simulink model "asbCubeSat"  (R2020a)
settings: Solver=ode3  StartTime=0.0  StopTime=86400*365.25*1  FixedStep=CubeSatTimeStep  RelTol=1e-3  EnableMultiTasking=on
PreLoadFcn:
  | if ~builtin('license','test','Virtual_Reality_Toolbox')
  |     assignin('base','variantVisualization',0)
  | end
PostLoadFcn:
  | ATM_Model=3 %
InitFcn:
  | if evalin('base', 'exist(''variantVisualization'',''var'')') && ...
  |         evalin('base', 'variantVisualization == 1')
  |     if ~builtin('license','checkout','Virtual_Reality_Toolbox')
  |         error(message('aeroblks_cubesat:cubesat:licenseFailAnim'));
  |     end
  | end
  | 
  | if ~evalin('base','exist(''CubeSatTimeStep'')')
  |     assignin('base','CubeSatTimeStep',1);
  | end
StopFcn:
  | %save('./work/simulation/alt_km_simulation.mat','alt_km_simulation','-v7.3')
  | 
  | save( ['./work/simulation/alt_km_simulation','_a_',get_param('asbCubeSat/Edit Initial Orbit and Attitude', 'a'), '_Area_', sprintf('%.4f',vehicle.Area),'.mat'],'alt_km_simulation','-v7.3')
undefined symbols (not defined in the file): CubeSatTimeStep, initCond, magnitude, Solar_Activity, vehicle
libraries: aerolibutil x12, aerolibatmos2 x6, aerolibconvert2 x3, simulink x2, asbCubeSatEnvironmentLib x1, SignalEditorBlockLib x1, sharedutil x1, asbCubeSatActuatorsLib x1, asbCubeSatSensorsLib x1, asbCubeSatDynamicsLib x1, asbCubeSatFSWLib x1, aerolibobsolete x1
(part 1 of 2)
settings Model: RequirementInfo={} %GIDa_aedc6be2_fb6a_446c_8c25_10b8bc9db182  SimulationMode=accelerator  SnapshotInterval=1  ExtModeAutoUpdateStatusClock=off  OrderedModelArguments=off  Creator=The MathWorks, Inc.  LastModifiedBy=ge49gar
settings SolverCC: AutoInsertRateTranBlk=on
settings DataIOCC: LimitDataPoints=on  SaveFormat=Array  SaveOutput=off  DSMLogging=off  SaveTime=off  ReturnWorkspaceOutputs=off
settings OptimizationCC: DefaultParameterBehavior=Inlined  OptimizeBlockIOStorage=off  BufferReuse=off  GlobalBufferReuse=off  ExpressionFolding=off  ExpressionDepthLimit=2147483647  LocalBlockOutputs=off  InitFltsAndDblsToZero=on  LifeSpan=inf  OptimizeDataStoreBuffers=off  BusAssignmentInplaceUpdate=off
settings DebuggingCC: SignalResolutionControl=TryResolveAllWithWarning  MultiTaskDSMMsg=warning  MultiTaskCondExecSysMsg=none  AssertControl=DisableAll  StateNameClashWarn=warning  PregeneratedLibrarySubsystemCodeDiagnostic=none  SFUnexpectedBacktrackingDiag=warning  SFNoUnconditionalDefaultTransitionDiag=warning  SFExecutionAtInitializationDiag=none  ArithmeticOperatorsInVariantConditions=warning
settings HardwareCC: ProdBitPerPointer=32  ProdBitPerSizeT=32  ProdBitPerPtrDiffT=32  ProdLargestAtomicFloat=None  ProdIntDivRoundTo=Undefined  ProdEndianess=Unspecified  ProdWordSize=32  ProdHWDeviceType=32-bit Generic
settings ModelReferenceCC: UpdateModelReferenceTargets=IfOutOfDate  ModelReferenceMinAlgLoopOccurrences=on  PropagateSignalLabelsOutOfModel=off
settings SFSimCC: SimUseLocalCustomCode=off
settings RTWCC: RTWUseLocalCustomCode=off
settings CodeAppCC: StateflowObjectComments=on
settings GRTTargetCC: TargetFcnLib=ansi_tfl_tmw.mat  TargetLangStandard=C89/C90 (ANSI)  CombineOutputUpdateFcns=off  GRTInterface=on
settings ConfigComp: CovMetricSettings=dw  CovHtmlReporting=on  CovSaveCumulativeToWorkspaceVar=on  CovSaveSingleToWorkspaceVar=on  CovExternalEMLEnable=off

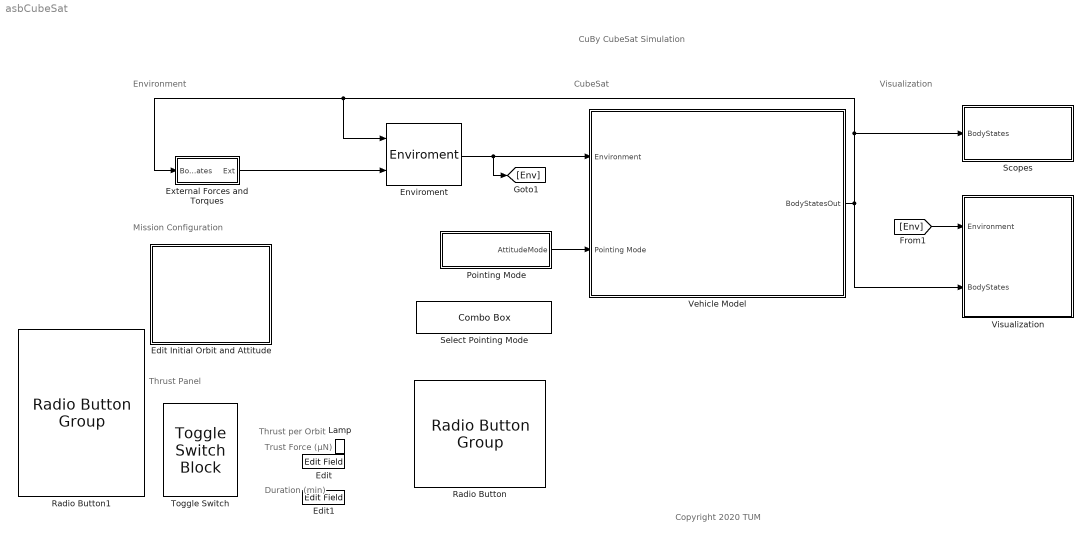
== system asbCubeSat ==
  note: Duration (min)
  note: Trust Force (µN)
  note: Thrust per Orbit
  note: Thrust Panel
  note: Visualization
  note: CubeSat
  note: Environment
  note: Copyright 2020 TUM
  note: CuBy CubeSat Simulation
  note: Mission Configuration
  Edit : EditField  LabelPosition=Hide  ShowInitialText=on  Alignment=Center
  Edit Initial Orbit and Attitude : Subsystem  mask(CubeSat Initial Conditions){sim_t0=2458928.8744, epoch=2452637.5, method=Keplerian Orbital Elements, a=6740285, ecc=0.1, incl=96.89, omega=337.5, argp=93.4872, nu=302.9234, truelon=0, arglat=0, lonper=0, r_eci=[4533222.8936 -2365511.728 3729499.3489], v_eci=[-5234.4767 1366.6412 6128.4254], r_ecef=[4811340.466 1709232.8008 3739578.4636], v_ecef=[-4446.0927 -3269.5147 6116.7671], lla=[36.4038927 19.5576255 -41750.4973], v_ned=[8059.0526 -1592.5303 622.75621], euler=[0 0 0], pqr=[0 0 -0.05168], dAT=37, dUT1=-0.1193, pm=[2.141e-05 6.93e-05], dCIP=[1.014e-07 -6.81e-08], lod=0}
      mask prompts: sim_t0 "aeroblks_cubesat:cubesat:StartDate"; epoch "aeroblks_cubesat:cubesat:ECIEpoch"; method "aeroblks_cubesat:cubesat:InputMethod"; a "aeroblks_cubesat:cubesat:SemiMajorAxis"; ecc "aeroblks_cubesat:cubesat:Eccentricity"; incl "aeroblks_cubesat:cubesat:Inclination"; omega "aeroblks_cubesat:cubesat:RAAN"; argp "aeroblks_cubesat:cubesat:ArgP"; nu "aeroblks_cubesat:cubesat:TrueAnomaly"; truelon "aeroblks_cubesat:cubesat:TrueLon"; arglat "aeroblks_cubesat:cubesat:ArgLat"; lonper "aeroblks_cubesat:cubesat:LonPer"; r_eci "aeroblks_cubesat:cubesat:ECIPos"; v_eci "aeroblks_cubesat:cubesat:ECIVel"; r_ecef "aeroblks_cubesat:cubesat:ECEFPos"; v_ecef "aeroblks_cubesat:cubesat:ECEFVel"; lla "aeroblks_cubesat:cubesat:LLA"; v_ned "aeroblks_cubesat:cubesat:NEDVel"; euler "aeroblks_cubesat:cubesat:Euler"; pqr "aeroblks_cubesat:cubesat:BodyAngRates"; dAT "aeroblks_cubesat:cubesat:dTAI"; dUT1 "aeroblks_cubesat:cubesat:DUT1"; pm "aeroblks_cubesat:cubesat:DPolar"; dCIP "aeroblks_cubesat:cubesat:DCIP"; lod "aeroblks_cubesat:cubesat:DLOD"
      mask help: aeroblks_cubesat:cubesat:InitCondBlockDesc
      mask init:
      | initCond = cubeSatCallback(gcb, 'computeIC', method, sim_t0, epoch, a, ecc, incl,...
      |     omega, argp, nu, truelon, arglat, lonper, r_eci, v_eci, r_ecef, v_ecef, lla,...
      |     v_ned, euler, pqr, dAT, dUT1, pm, dCIP, lod);
      mask TypeOptions method: aeroblks_cubesat:cubesat:InputKeplerian | aeroblks_cubesat:cubesat:InputECI | aeroblks_cubesat:cubesat:InputECEF | aeroblks_cubesat:cubesat:InputLLANED
      mask Callback method: cubeSatCallback(gcb, 'handleMethod');
      mask Callback ecc: cubeSatCallback(gcb, 'handleCircularOrbit');
      mask Callback incl: cubeSatCallback(gcb, 'handleCircularOrbit');
      mask DialogControl sim_t0 Prompt: Start date [Julian date]:
      mask DialogControl sim_t0 Tooltip: aeroblks_cubesat:cubesat:StartDateTT
      mask DialogControl icTab Prompt: aeroblks_cubesat:cubesat:InitCond
      mask DialogControl epoch Prompt: Epoch of ECI frame [Julian date]:
      mask DialogControl epoch Tooltip: aeroblks_cubesat:cubesat:ECIEpochTT
      mask DialogControl Container9 Prompt: aeroblks_cubesat:cubesat:InitCondOrbit
      mask DialogControl method Prompt: Input method:
      mask DialogControl method Tooltip: aeroblks_cubesat:cubesat:InputMethodTT
      mask DialogControl a Prompt: Semi-major axis [m]:
      mask DialogControl a Tooltip: aeroblks_cubesat:cubesat:SemiMajorAxisTT
      mask DialogControl ecc Prompt: Eccentricity:
      mask DialogControl ecc Tooltip: aeroblks_cubesat:cubesat:EccentricityTT
      mask DialogControl incl Prompt: Inclination [deg]:
      mask DialogControl incl Tooltip: aeroblks_cubesat:cubesat:InclinationTT
      mask DialogControl omega Prompt: Right ascension of the ascending node [deg]:
      mask DialogControl omega Tooltip: aeroblks_cubesat:cubesat:RAANTT
      mask DialogControl argp Prompt: Argument of periapsis [deg]:
      mask DialogControl argp Tooltip: aeroblks_cubesat:cubesat:ArgPTT
      mask DialogControl nu Prompt: True anomaly [deg]:
      mask DialogControl nu Tooltip: aeroblks_cubesat:cubesat:TrueAnomalyTT
      mask DialogControl truelon Prompt: True longitude [deg] (circular equatorial):
      mask DialogControl truelon Tooltip: aeroblks_cubesat:cubesat:TrueLonTT
      mask DialogControl arglat Prompt: Argument of latitude [deg] (circular inclined):
      mask DialogControl arglat Tooltip: aeroblks_cubesat:cubesat:ArgLatTT
      mask DialogControl lonper Prompt: Longitude of periapsis [deg] (elliptical equatorial):
      mask DialogControl lonper Tooltip: aeroblks_cubesat:cubesat:LonPerTT
      mask DialogControl r_eci Prompt: ECI position vector [m]:
      mask DialogControl r_eci Tooltip: aeroblks_cubesat:cubesat:ECIPosTT
      mask DialogControl v_eci Prompt: ECI velocity vector [m/s]:
      mask DialogControl v_eci Tooltip: aeroblks_cubesat:cubesat:ECIVelTT
      mask DialogControl r_ecef Prompt: ECEF position vector [m]:
      mask DialogControl r_ecef Tooltip: aeroblks_cubesat:cubesat:ECEFPosTT
      mask DialogControl v_ecef Prompt: ECEF velocity vector [m/s]:
      mask DialogControl v_ecef Tooltip: aeroblks_cubesat:cubesat:ECEFVelTT
      mask DialogControl lla Prompt: Geodetic latitude, longitude, altitude [deg, deg, m]:
      mask DialogControl lla Tooltip: aeroblks_cubesat:cubesat:LLATT
      mask DialogControl v_ned Prompt: NED velocity vector [m/s]:
      mask DialogControl v_ned Tooltip: aeroblks_cubesat:cubesat:NEDVelTT
      mask DialogControl Container11 Prompt: aeroblks_cubesat:cubesat:InitCondAttitude
      mask DialogControl euler Prompt: <html>Initial Euler angles (roll, pitch, yaw) [deg]:</html>
      mask DialogControl euler Tooltip: aeroblks_cubesat:cubesat:EulerTT
      mask DialogControl pqr Prompt: Initial body angular rates [deg/s]:
      mask DialogControl pqr Tooltip: aeroblks_cubesat:cubesat:BodyAngRatesTT
      mask DialogControl epTab Prompt: aeroblks_cubesat:cubesat:EOPTab
      mask DialogControl dAT Prompt: Difference between TAI and UTC [sec]:
      mask DialogControl dAT Tooltip: aeroblks_cubesat:cubesat:dTAITT
      mask DialogControl dUT1 Prompt: Difference between UTC and UT1 [sec]:
      mask DialogControl dUT1 Tooltip: aeroblks_cubesat:cubesat:DUT1TT
      mask DialogControl pm Prompt: Polar displacement [deg deg]:
      mask DialogControl pm Tooltip: aeroblks_cubesat:cubesat:DPolarTT
      mask DialogControl dCIP Prompt: CIP adjustment [deg deg]:
      mask DialogControl dCIP Tooltip: aeroblks_cubesat:cubesat:DCIPTT
      mask DialogControl lod Prompt: Excess length of day [sec]:
      mask DialogControl lod Tooltip: aeroblks_cubesat:cubesat:DLODTT
      mask Display:
      | text(.1, .9, [' a = ' sprintf('%.1f', str2double(get_param(gcb, 'a'))) ' m'],'horizontalAlignment','left','texmode','on');
      | text(.1, .75, [' e = ' get_param(gcb, 'ecc')],'horizontalAlignment','left','texmode', 'on')
      | text(.1, .6, ['  i = ' get_param(gcb, 'incl') '\circ'],'horizontalAlignment','left','texmode', 'on')
      | text(.1, .45, ['\Omega = ' get_param(gcb, 'omega') '\circ'],'horizontalAlignment','left','texmode', 'on')
      | text(.1, .3, ['\omega = ' get_param(gcb, 'argp') '\circ'],'horizontalAlignment','left','texmode', 'on')
      | text(.1, .15, [' \nu = ' get_param(gcb, 'nu') '\circ'],'horizontalAlignment','left','texmode', 'on')
  Edit1 : EditField  LabelPosition=Hide  ShowInitialText=on  Alignment=Center
  Enviroment : asbCubeSatEnvironmentLib/Enviroment  SystemSampleTime=-1  Latency=0  AutoFrameSizeCalculation=off
  External Forces and Torques : Subsystem
  Lamp : LampBlock  LabelPosition=Hide
  Pointing Mode : Subsystem
  Radio Button : RadioButtonGroup  LabelPosition=Hide  SelectedLabel=NRLMSISE-00 + F10.7 & Ap  ButtonGroupName=Atmospheric Model
      settings: Values={{'No Drag', 'ISA', 'NRLMSISE-00', 'NRLMSISE-00 + F10.7 & Ap'}, [0 1 2 3]}
  Radio Button1 : RadioButtonGroup  ButtonGroupName=Group
      settings: Values={{'Label1', 'Label2', 'Label3'}, [0 1 2]}
  Scopes : Subsystem  VariantControl=visOff
  Select Pointing Mode : ComboBox  LabelPosition=Hide  SelectedLabel=Nadir Pointing (Earth)
      settings: Values={{'Standby', 'Nadir Pointing (Earth)', 'Sun Tracking', 'Custom Schedule'}, [0 1 2 3]}
  Toggle Switch : ToggleSwitchBlock
      settings: Values={{'Off', 'On'}, [0 1]}
  Vehicle Model : Subsystem
      mask Display: image('CubeSatVehicle.PNG');
  Visualization : Subsystem  Variant=on  mask(Set Animation Properties){visSampleTime=5, cubesatSize=2e5, showAntenna=on, antennaHeight=1e6, antennaHalfAngle=25}
      mask prompts: visSampleTime "aeroblks_cubesat:cubesat:AnimSampleTime"; cubesatSize "aeroblks_cubesat:cubesat:MdlSize"; showAntenna "aeroblks_cubesat:cubesat:ShowCone"; antennaHeight "aeroblks_cubesat:cubesat:ConeHeight"; antennaHalfAngle "aeroblks_cubesat:cubesat:ConeAngle"
      mask help: aeroblks_cubesat:cubesat:VisBlockDesc
      mask Callback showAntenna:
      | if evalin('base', 'exist(''variantVisualization'',''var'')') ...
      |     && evalin('base', 'variantVisualization == 1') ...
      |     && builtin('license','test','Virtual_Reality_Toolbox')
      | 
      |     enable = get_param(gcb,'MaskEnables');
      |     if strcmp(get_param(gcb, 'showAntenna'), 'off')
      |         enable(4:5) = {'off'};
      |     else
      |         enable(4:5) = {'on'};
      |     end
      |     set_param(gcb,'MaskEnables', enable);
      |     clear enable
      | end
      mask DialogControl vrOpenBtn Prompt: aeroblks_cubesat:cubesat:AnimOpenBtn
      mask DialogControl vrOpenBtn Callback:
      | if builtin('license','checkout','Virtual_Reality_Toolbox')
      |     vrmfunc('FnOpen',getSimulinkBlockHandle([gcb '/Virtual Reality World/VR Sink']));
      | end
      mask DialogControl visSampleTime Prompt: Animation refresh rate:
      mask DialogControl visSampleTime Tooltip: aeroblks_cubesat:cubesat:AnimSampleTimeTT
      mask DialogControl cubesatSize Prompt: CubeSat display size [m]:
      mask DialogControl cubesatSize Tooltip: aeroblks_cubesat:cubesat:MdlSizeTT
      mask DialogControl Container3 Prompt: aeroblks_cubesat:cubesat:AntennaPropArea
      mask DialogControl showAntenna Prompt: Show antenna cone in animation
      mask DialogControl showAntenna Tooltip: aeroblks_cubesat:cubesat:ShowConeTT
      mask DialogControl antennaHeight Prompt: Antenna cone height [m]:
      mask DialogControl antennaHeight Tooltip: aeroblks_cubesat:cubesat:ConeHeightTT
      mask DialogControl antennaHalfAngle Prompt: Antenna cone half angle [deg]:
      mask DialogControl antennaHalfAngle Tooltip: aeroblks_cubesat:cubesat:ConeAngleTT
  wires:
  Enviroment/1 -> [Env], Vehicle Model/1(Environment)
  External Forces and Torques/1(Ext) -> Enviroment/2
  Vehicle Model/1(BodyStatesOut) -> Visualization/2(BodyStates), Scopes/1(BodyStates), External Forces and Torques/1(BodyStates), Enviroment/1
  Pointing Mode/1(AttitudeMode) -> Vehicle Model/2(Pointing Mode)
  [Env] -> Visualization/1(Environment)

== system asbCubeSat/Edit Initial Orbit and Attitude ==

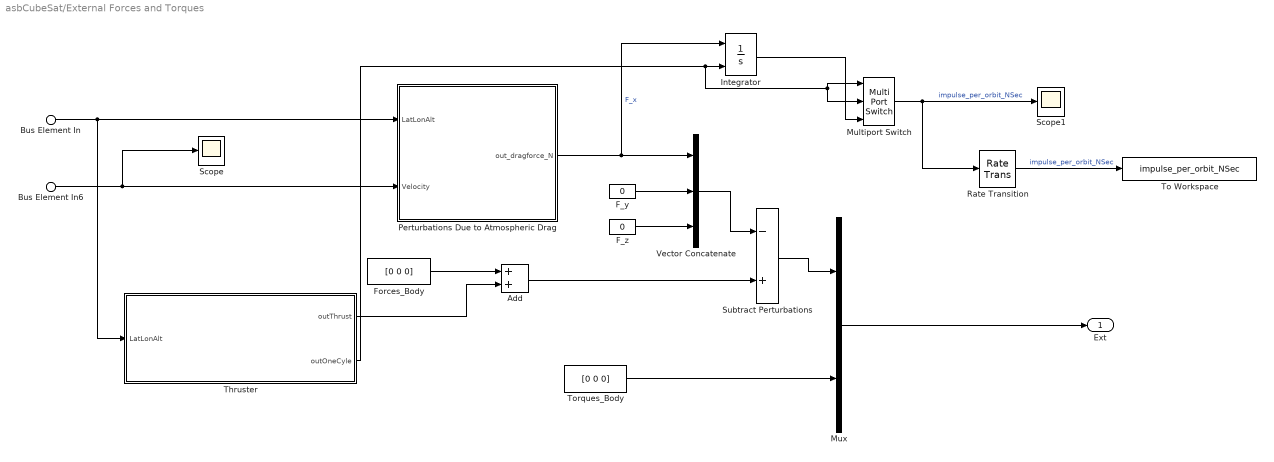
== system asbCubeSat/External Forces and Torques ==
  Bus Element In : Inport  PortName=BodyStates  Element=LatLonAlt
  Bus Element In6 : Inport  PortName=BodyStates  Element=V_ecef
  Add : Sum
  F_y : Constant  Value=0
  F_z : Constant  Value=0
  Forces_Body : Constant  Value=[0 0 0]
  Integrator : Integrator  ExternalReset=falling
  Multiport Switch : MultiPortSwitch  DataPortOrder=Zero-based contiguous  Inputs=2  zeroidx=on
  Mux : Mux  RequirementInfo={} %GIDa_ef4ca723_4eef_40f8_bb1e_99de60d2b248  Inputs=2
  Perturbations Due to Atmospheric Drag : Subsystem
  Rate Transition : RateTransition  OutPortSampleTime=60
  Scope : Scope
  Scope1 : Scope
  "Subtract Perturbations " : Sum  Inputs=-+
  Thruster : Subsystem
  To Workspace : ToWorkspace  VariableName=impulse_per_orbit_NSec  SaveFormat=Structure With Time  SampleTime=-1
  Torques_Body : Constant  Value=[0 0 0]
  Vector Concatenate : Concatenate  NumInputs=3
  Ext : Outport  RequirementInfo={} %GIDa_0f078eca_6127_499d_b81c_658503a40261  VectorParamsAs1DForOutWhenUnconnected=off
  wires:
  Forces_Body/1 -> Add/1
  Torques_Body/1 -> Mux/2
  Mux/1 -> Ext/1
  "Subtract Perturbations "/1 -> Mux/1
  Perturbations Due to Atmospheric Drag/1(out_dragforce_N) -> Integrator/1, Vector Concatenate/1  "F_x"
  Vector Concatenate/1 -> "Subtract Perturbations "/1
  F_y/1 -> Vector Concatenate/2
  F_z/1 -> Vector Concatenate/3
  Bus Element In/1 -> Thruster/1(LatLonAlt), Perturbations Due to Atmospheric Drag/1(LatLonAlt)
  Bus Element In6/1 -> Scope/1, Perturbations Due to Atmospheric Drag/2(Velocity)
  Thruster/1(outThrust) -> Add/2
  Add/1 -> "Subtract Perturbations "/2
  Thruster/2(outOneCyle) -> Multiport Switch/2, Multiport Switch/1, Integrator/2
  Integrator/1 -> Multiport Switch/3
  Multiport Switch/1 -> Scope1/1, Rate Transition/1  "impulse_per_orbit_NSec"
  Rate Transition/1 -> To Workspace/1  "impulse_per_orbit_NSec"

== system asbCubeSat/Pointing Mode ==
  note: Modes:
      | 0 = Off
      | 1 = Earth (Nadir)
      | 2 = Sun
  Mode : Constant  SampleTime=-1
  Multiport Switch : MultiPortSwitch  DataPortOrder=Specify indices  DataPortIndices={3, [0,1,2]}  DiagnosticForDefault=None
  Signal Editor : SignalEditorBlockLib/Signal Editor  FileName=SignalEditorPointing.mat  ActiveScenario=PointingScenario  ActiveSignal=PointingMode  IsBus=off  OutputBusObjectStr=Bus: BusObject  SampleTime=0  Interpolate=off  ZeroCross=off  OutputAfterFinalValue=Setting to zero  Unit=inherit  PreserveSignalName=on
  AttitudeMode : Outport  VectorParamsAs1DForOutWhenUnconnected=off
  wires:
  Signal Editor/1 -> Multiport Switch/2
  Mode/1 -> Multiport Switch/1, Multiport Switch/3
  Multiport Switch/1 -> AttitudeMode/1

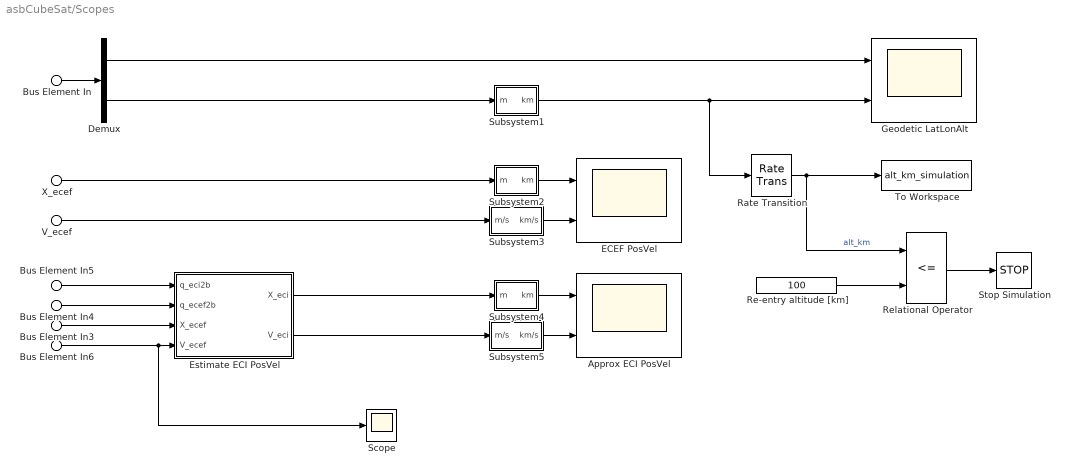
== system asbCubeSat/Scopes ==
  Bus Element In : Inport  PortName=BodyStates  Element=LatLonAlt
  X_ecef : Inport  PortName=BodyStates  Element=X_ecef
  Bus Element In3 : Inport  PortName=BodyStates  Element=X_ecef
  V_ecef : Inport  PortName=BodyStates  Element=V_ecef
  Bus Element In6 : Inport  PortName=BodyStates  Element=V_ecef
  Bus Element In4 : Inport  PortName=BodyStates  Element=q_ecef2b
  Bus Element In5 : Inport  PortName=BodyStates  Element=q_eci2b
  Approx ECI PosVel : Scope  NumInputPorts=2
  Demux : Demux  Outputs=[2 1]
  ECEF PosVel : Scope  NumInputPorts=2
  Estimate ECI PosVel : Subsystem
  Geodetic LatLonAlt : Scope  NumInputPorts=2
  Rate Transition : RateTransition  OutPortSampleTime=60
  Re-entry altitude [km] : Constant  Value=100
  Relational Operator : RelationalOperator  Operator=<=  OutDataTypeStr=boolean  RndMeth=Simplest
  Scope : Scope
  Stop Simulation : Stop
  Subsystem1 : Subsystem
  Subsystem2 : Subsystem
  Subsystem3 : Subsystem
  Subsystem4 : Subsystem
  Subsystem5 : Subsystem
  To Workspace : ToWorkspace  VariableName=alt_km_simulation  SaveFormat=Structure With Time  SampleTime=-1
  wires:
  Bus Element In/1 -> Demux/1
  Demux/1 -> Geodetic LatLonAlt/1
  Demux/2 -> Subsystem1/1(m)
  X_ecef/1 -> Subsystem2/1(m)
  V_ecef/1 -> Subsystem3/1(m/s)
  Estimate ECI PosVel/1(X_eci) -> Subsystem4/1(m)
  Estimate ECI PosVel/2(V_eci) -> Subsystem5/1(m/s)
  Bus Element In5/1 -> Estimate ECI PosVel/1(q_eci2b)
  Bus Element In4/1 -> Estimate ECI PosVel/2(q_ecef2b)
  Bus Element In3/1 -> Estimate ECI PosVel/3(X_ecef)
  Subsystem1/1(km) -> Rate Transition/1, Geodetic LatLonAlt/2
  Subsystem2/1(km) -> ECEF PosVel/1
  Subsystem3/1(km/s) -> ECEF PosVel/2
  Subsystem4/1(km) -> Approx ECI PosVel/1
  Subsystem5/1(km/s) -> Approx ECI PosVel/2
  Bus Element In6/1 -> Scope/1, Estimate ECI PosVel/4(V_ecef)
  Rate Transition/1 -> Relational Operator/1, To Workspace/1  "alt_km"
  Relational Operator/1 -> Stop Simulation/1
  Re-entry altitude [km]/1 -> Relational Operator/2

== system asbCubeSat/Vehicle Model ==
  note: Flight Software
  note: Plant Model
  Environment : Inport
  Pointing Mode : Inport  Port=2
  Vehicle Control Actuators : asbCubeSatActuatorsLib/Vehicle Control Actuators  SystemSampleTime=-1  Latency=0  AutoFrameSizeCalculation=off
  Vehicle Control Sensors : asbCubeSatSensorsLib/Vehicle Control Sensors  SystemSampleTime=-1  Latency=0  AutoFrameSizeCalculation=off
  Vehicle Dynamics : asbCubeSatDynamicsLib/Vehicle Dynamics  SystemSampleTime=-1  Latency=0  AutoFrameSizeCalculation=off
  Vehicle Flight Software : asbCubeSatFSWLib/Vehicle Flight Software  SystemSampleTime=-1  Latency=0  AutoFrameSizeCalculation=off
  BodyStatesOut : Outport  OutDataTypeStr=Bus: StatesOutBus  VectorParamsAs1DForOutWhenUnconnected=off
  wires:
  Vehicle Dynamics/1 -> Vehicle Control Sensors/1, BodyStatesOut/1
  Pointing Mode/1 -> Vehicle Flight Software/1
  Vehicle Control Sensors/1 -> Vehicle Flight Software/3
  Vehicle Control Actuators/1 -> Vehicle Dynamics/1
  Vehicle Control Actuators/2 -> Vehicle Dynamics/2
  Vehicle Flight Software/1 -> Vehicle Control Actuators/1
  Environment/1 -> Vehicle Dynamics/3, Vehicle Flight Software/2

== system asbCubeSat/Visualization ==
  Environment : Inport
  BodyStates : Inport  RequirementInfo={} %GIDa_d1e0371a_f352_4707_a071_6ff04189e700  Port=2
  No Visualization : Subsystem  VariantControl=visOff
  Virtual Reality World : Subsystem  VariantControl=visSL3D

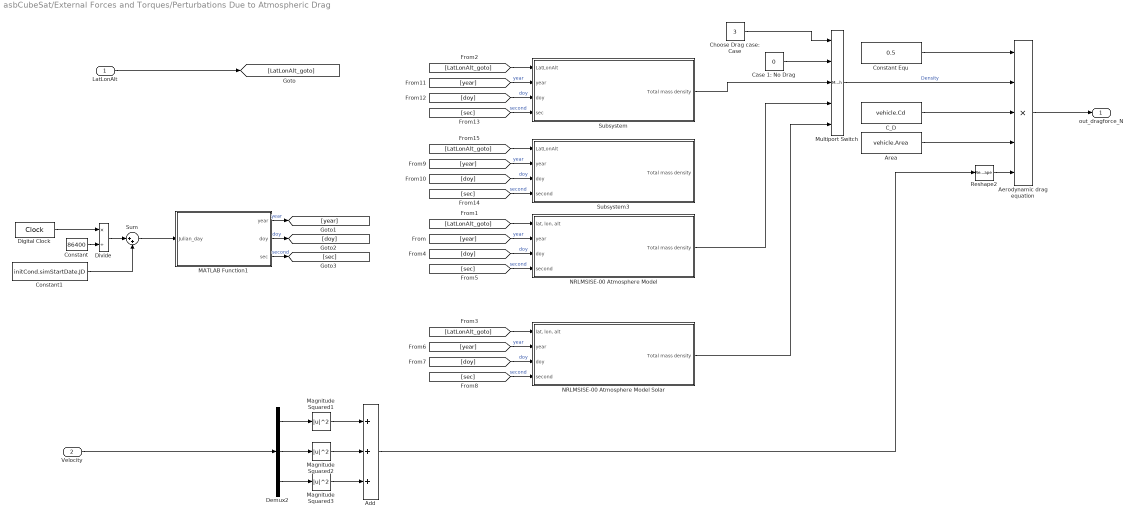
== system asbCubeSat/External Forces and Torques/Perturbations Due to Atmospheric Drag ==
  LatLonAlt : Inport
  Velocity : Inport  Port=2
  Add : Sum  Inputs=3
  Aerodynamic drag equation : Product  Inputs=*****
  Area : Constant  Value=vehicle.Area
  C_D : Constant  Value=vehicle.Cd
  Case 1: No Drag : Constant  Value=0
  Choose Drag case: Case : Constant  Value=3
  Constant : Constant  Value=86400
  Constant Equ : Constant  Value=0.5
  Constant1 : Constant  Value=initCond.simStartDate.JD
  Demux2 : Demux  Outputs=3
  Digital Clock : DigitalClock  SampleTime=CubeSatTimeStep
  Divide : Product  Inputs=*/
  MATLAB Function1 : MATLAB Function  TreatAsAtomicUnit=on
  Magnitude Squared1 : Math  Operator=magnitude^2  SaturateOnIntegerOverflow=on
  Magnitude Squared2 : Math  Operator=magnitude^2  SaturateOnIntegerOverflow=on
  Magnitude Squared3 : Math  Operator=magnitude^2  SaturateOnIntegerOverflow=on
  Multiport Switch : MultiPortSwitch  DataPortOrder=Zero-based contiguous  Inputs=4  zeroidx=on
  NRLMSISE-00 Atmosphere Model : Subsystem
  NRLMSISE-00 Atmosphere Model Solar : Subsystem
  Reshape2 : Reshape
  Subsystem : Subsystem
  Subsystem3 : Subsystem  StartFcn=set_param(gcb,'asbCubeSat/External Forces and Torques /Perturbations Due to Atmospheric Drag/Choose Drag case: Case','Value'));  Variant=on  VariantControlMode=Label  VariantControl=Choice  LabelModeActiveChoice=3  PropagateVariantConditions=on  mask{ChooseModel=3}
      mask prompts: ChooseModel "Choose variant:"
      mask TypeOptions ChooseModel: 0 | 1 | 2 | 3
      mask Callback ChooseModel:
      | set_param(gcb,'OverrideUsingVariant',(get_param('asbCubeSat/External Forces and Torques/Perturbations Due to Atmospheric Drag/Choose Drag case: Case', 'Value')));
      | set_param(gcb, 'ChooseModel', get_param('asbCubeSat/External Forces and Torques/Perturbations Due to Atmospheric Drag/Choose Drag case: Case', 'Value'));
  Sum : Sum  Inputs=|++
  out_dragforce_N : Outport
  wires:
  LatLonAlt/1 -> [LatLonAlt_goto]
  Case 1: No Drag/1 -> Multiport Switch/2
  Choose Drag case: Case/1 -> Multiport Switch/1
  Constant Equ/1 -> Aerodynamic drag equation/1
  C_D/1 -> Aerodynamic drag equation/3
  Area/1 -> Aerodynamic drag equation/4
  Multiport Switch/1 -> Aerodynamic drag equation/2  "Density"
  Aerodynamic drag equation/1 -> out_dragforce_N/1
  Add/1 -> Reshape2/1
  Reshape2/1 -> Aerodynamic drag equation/5
  Magnitude Squared3/1 -> Add/3
  Demux2/3 -> Magnitude Squared3/1
  Demux2/1 -> Magnitude Squared1/1
  Demux2/2 -> Magnitude Squared2/1
  Magnitude Squared1/1 -> Add/1
  Magnitude Squared2/1 -> Add/2
  Velocity/1 -> Demux2/1
  Constant1/1 -> Sum/2
  Divide/1 -> Sum/1
  Digital Clock/1 -> Divide/1
  Sum/1 -> MATLAB Function1/1(Julian_day)
  Constant/1 -> Divide/2
  MATLAB Function1/3(sec) -> [sec]  "second"
  MATLAB Function1/2(doy) -> [doy]  "doy"
  MATLAB Function1/1(year) -> [year]  "year"
  [LatLonAlt_goto] -> NRLMSISE-00 Atmosphere Model Solar/1("lat, lon, alt")
  [year] -> NRLMSISE-00 Atmosphere Model Solar/2(year)  "year"
  [doy] -> NRLMSISE-00 Atmosphere Model Solar/3(doy)  "doy"
  [sec] -> NRLMSISE-00 Atmosphere Model Solar/4(second)  "second"
  NRLMSISE-00 Atmosphere Model Solar/1(Total mass density) -> Multiport Switch/5
  [LatLonAlt_goto] -> NRLMSISE-00 Atmosphere Model/1("lat, lon, alt")
  [year] -> NRLMSISE-00 Atmosphere Model/2(year)  "year"
  [doy] -> NRLMSISE-00 Atmosphere Model/3(doy)  "doy"
  [sec] -> NRLMSISE-00 Atmosphere Model/4(second)  "second"
  NRLMSISE-00 Atmosphere Model/1(Total mass density) -> Multiport Switch/4
  [LatLonAlt_goto] -> Subsystem/1(LatLonAlt)
  Subsystem/1(Total mass density) -> Multiport Switch/3
  [year] -> Subsystem/2(year)  "year"
  [doy] -> Subsystem/3(doy)  "doy"
  [sec] -> Subsystem/4(sec)  "second"
  [LatLonAlt_goto] -> Subsystem3/1(LatLonAlt)
  [year] -> Subsystem3/2(year)  "year"
  [doy] -> Subsystem3/3(doy)  "doy"
  [sec] -> Subsystem3/4(second)  "second"

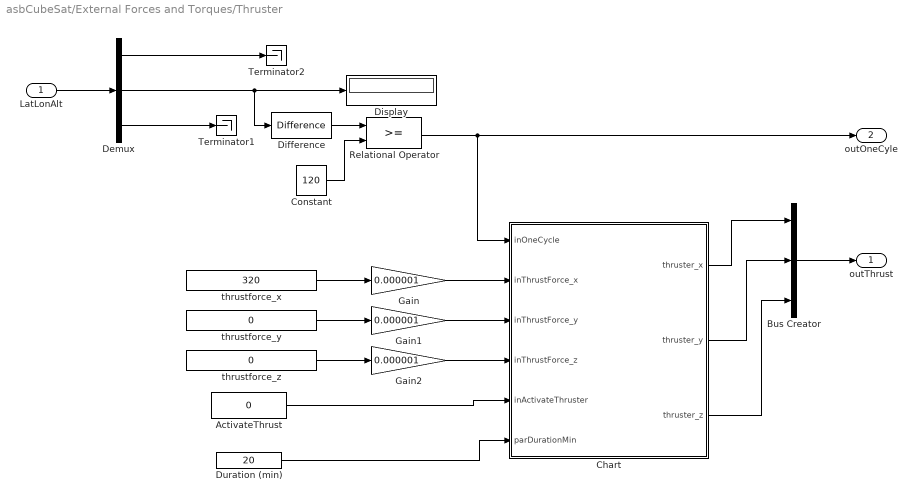
== system asbCubeSat/External Forces and Torques/Thruster ==
  LatLonAlt : Inport
  ActivateThrust : Constant  Value=0
  Bus Creator : BusCreator  Inputs=3
  Chart : Stateflow chart  TreatAsAtomicUnit=on
  Constant : Constant  Value=120
  Demux : Demux  Outputs=3
  Difference : simulink/Discrete/Difference  ICPrevInput=0.0  OutMin=[]  OutMax=[]  OutDataType=fixdt(1, 16)  OutScaling=2^-10  DoSatur=off
  Display : Display
  Duration (min) : Constant  Value=20
  Gain : Gain  Gain=0.000001
  Gain1 : Gain  Gain=0.000001
  Gain2 : Gain  Gain=0.000001
  Relational Operator : RelationalOperator  OutDataTypeStr=boolean  RndMeth=Simplest
  Terminator1 : Terminator
  Terminator2 : Terminator
  thrustforce_x : Constant  Value=320
  thrustforce_y : Constant  Value=0
  thrustforce_z : Constant  Value=0
  outThrust : Outport
  outOneCyle : Outport  Port=2
  wires:
  Demux/1 -> Terminator2/1
  Chart/3(thruster_z) -> Bus Creator/3
  Demux/3 -> Terminator1/1
  Chart/2(thruster_y) -> Bus Creator/2
  Constant/1 -> Relational Operator/2
  Chart/1(thruster_x) -> Bus Creator/1
  Demux/2 -> Display/1, Difference/1
  LatLonAlt/1 -> Demux/1
  Difference/1 -> Relational Operator/1
  Relational Operator/1 -> outOneCyle/1, Chart/1(inOneCycle)
  Bus Creator/1 -> outThrust/1
  thrustforce_x/1 -> Gain/1
  Gain/1 -> Chart/2(inThrustForce_x)
  thrustforce_y/1 -> Gain1/1
  thrustforce_z/1 -> Gain2/1
  Gain1/1 -> Chart/3(inThrustForce_y)
  Gain2/1 -> Chart/4(inThrustForce_z)
  ActivateThrust/1 -> Chart/5(inActivateThruster)
  Duration (min)/1 -> Chart/6(parDurationMin)

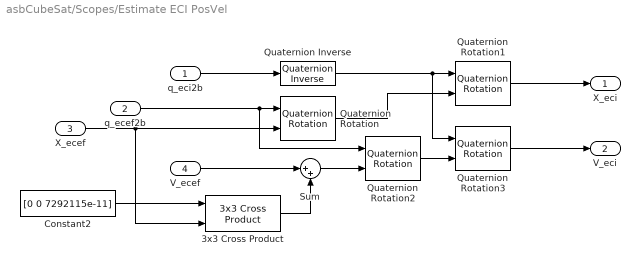
== system asbCubeSat/Scopes/Estimate ECI PosVel ==
  q_eci2b : Inport
  q_ecef2b : Inport  Port=2
  X_ecef : Inport  Port=3
  V_ecef : Inport  Port=4
  3x3 Cross Product : sharedutil/3x3 Cross Product  aMode=aMode
      settings: SourceProductBaseCode=AE,PW,MT,VE,VP
  Constant2 : Constant  RequirementInfo={} %GIDa_2ba99f61_3734_437b_bb66_1284a91b5056  Value=[0 0 7292115e-11]
  Quaternion Inverse : aerolibutil/Quaternion Inverse
  Quaternion Rotation{,1..3} (4 alike) : aerolibutil/Quaternion Rotation
  Sum : Sum  Inputs=|++
  X_eci : Outport  VectorParamsAs1DForOutWhenUnconnected=off
  V_eci : Outport  Port=2  VectorParamsAs1DForOutWhenUnconnected=off
  wires:
  Sum/1 -> Quaternion Rotation2/2
  3x3 Cross Product/1 -> Sum/2
  V_ecef/1 -> Sum/1
  Quaternion Rotation/1 -> Quaternion Rotation1/2
  q_ecef2b/1 -> Quaternion Rotation/1, Quaternion Rotation2/1
  Quaternion Inverse/1 -> Quaternion Rotation3/1, Quaternion Rotation1/1
  Constant2/1 -> 3x3 Cross Product/1
  Quaternion Rotation2/1 -> Quaternion Rotation3/2
  q_eci2b/1 -> Quaternion Inverse/1
  Quaternion Rotation1/1 -> X_eci/1
  X_ecef/1 -> 3x3 Cross Product/2, Quaternion Rotation/2
  Quaternion Rotation3/1 -> V_eci/1

== system asbCubeSat/Scopes/Subsystem1 ==
  m : Inport  Unit=m
  Unit Conversion : UnitConversion
  km : Outport  Unit=km  VectorParamsAs1DForOutWhenUnconnected=off
  wires:
  m/1 -> Unit Conversion/1
  Unit Conversion/1 -> km/1

== system asbCubeSat/Scopes/Subsystem2 ==
  m : Inport  Unit=m
  Unit Conversion : UnitConversion
  km : Outport  Unit=km  VectorParamsAs1DForOutWhenUnconnected=off
  wires:
  Unit Conversion/1 -> km/1
  m/1 -> Unit Conversion/1

== system asbCubeSat/Scopes/Subsystem3 ==
  m/s : Inport  Unit=m/s
  Unit Conversion : UnitConversion
  km/s : Outport  Unit=km/s  VectorParamsAs1DForOutWhenUnconnected=off
  wires:
  m/s/1 -> Unit Conversion/1
  Unit Conversion/1 -> km/s/1

== system asbCubeSat/Scopes/Subsystem4 ==
  m : Inport  Unit=m
  Unit Conversion : UnitConversion
  km : Outport  Unit=km  VectorParamsAs1DForOutWhenUnconnected=off
  wires:
  Unit Conversion/1 -> km/1
  m/1 -> Unit Conversion/1

== system asbCubeSat/Scopes/Subsystem5 ==
  m/s : Inport  Unit=m/s
  Unit Conversion : UnitConversion
  km/s : Outport  Unit=km/s  VectorParamsAs1DForOutWhenUnconnected=off
  wires:
  m/s/1 -> Unit Conversion/1
  Unit Conversion/1 -> km/s/1

== system asbCubeSat/Visualization/No Visualization ==
  BodyStates : Inport
  Environment : Inport  Port=2
  Terminator2 : Terminator
      settings: RequirementInfo={} %GIDa_803f6fff_5423_4e6f_a9df_7d3b0fb0a1d4
  Terminator3 : Terminator
      settings: RequirementInfo={} %GIDa_5d360e88_5b3d_45e7_ae99_5d46a57676c9
  wires:
  Environment/1 -> Terminator2/1
  BodyStates/1 -> Terminator3/1

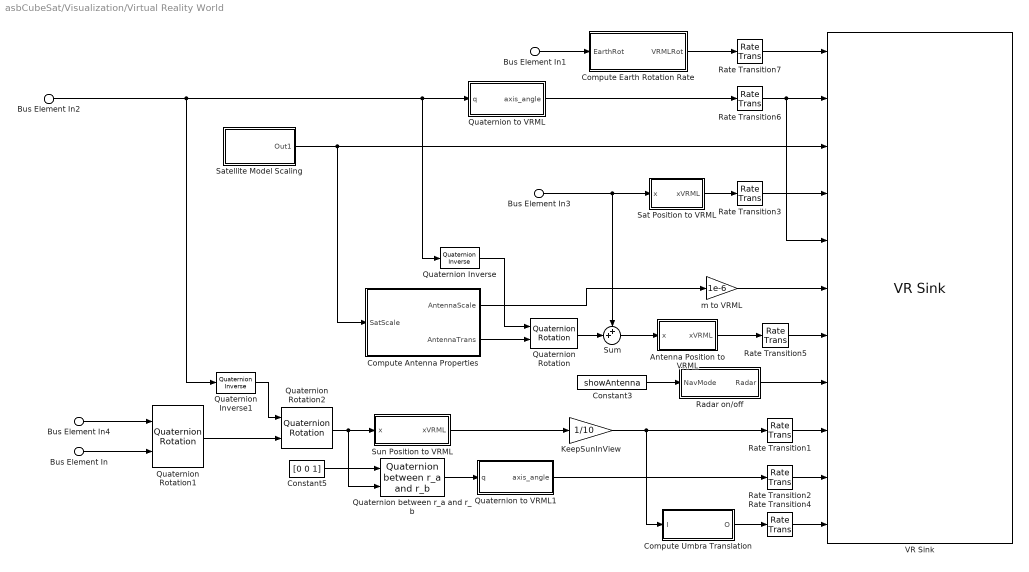
== system asbCubeSat/Visualization/Virtual Reality World ==
  Bus Element In3 : Inport  PortName=BodyStates  Element=X_ecef
  Bus Element In2 : Inport  PortName=BodyStates  Element=q_ecef2b
  Bus Element In4 : Inport  PortName=BodyStates  Element=q_eci2b
  Bus Element In : Inport  Port=2  PortName=Environment  Element=x_sun_eci
  Bus Element In1 : Inport  Port=2  PortName=Environment  Element=earthAngRate
  Antenna Position to VRML : Subsystem
  Compute Antenna Properties : Subsystem
  Compute Earth Rotation Rate : Subsystem
  Compute Umbra Translation : Subsystem
  Constant3 : Constant  Value=showAntenna
  Constant5 : Constant  Value=[0 0 1]
  KeepSunInView : Gain  Gain=1/10
  Quaternion Inverse : aerolibutil/Quaternion Inverse
  Quaternion Inverse1 : aerolibutil/Quaternion Inverse
  Quaternion Rotation : aerolibutil/Quaternion Rotation
  Quaternion Rotation1 : aerolibutil/Quaternion Rotation
  Quaternion Rotation2 : aerolibutil/Quaternion Rotation
  Quaternion between r_a and r_b : asbCubeSatBlockLib/Axes Transformations/Attitude Conversion/Quaternion between r_a and r_b  SystemSampleTime=-1  Latency=0  AutoFrameSizeCalculation=off
      settings: SourceProductBaseCode=AERO_CUBESAT
  Quaternion to VRML : Subsystem
  Quaternion to VRML1 : Subsystem
  Radar on/off : Subsystem
  Rate Transition{1..7} (7 alike) : RateTransition
  Sat Position to VRML : Subsystem
  Satellite Model Scaling : Subsystem
  Sum : Sum  Inputs=++|
  Sun Position to VRML : Subsystem
  VR Sink : vrlib/VR Sink  InstantiateOnLoad=on  SampleTime=visSampleTime  ViewEnable=on  RemoteChange=off  RemoteView=off  FieldsWritten=Earth.rotation.4.1.1.double#Satellite.rotation.4.1.1.double#Satellite.scale.3.1.1.double#Satellite.translation.3.1.1.double#AntennaCone.rotation.4.1.1.double#AntennaCone.scale.3.1.1.double#AntennaCone.translation.3.1.1.double#AntennaMaterial.transparency.1.1.1.double#Sun.translation.3.1.1.double#Umbra.rotation.4.1.1.double#Umbra.translation.3.1.1.double  WorldFileName=cubesatAnim.wrl  WorldDescription=CubeSat Orbit Animation  AutoView=on  VideoDimensions=[]  AllowVariableSize=off  FigureProperties="{'Position', 'Name', 'Viewpoint', 'CameraBound', 'CameraDirection', 'CameraPosition', 'CameraUpVector', 'ZoomFactor', 'Antialiasing', 'Headlight', 'Lighting', 'NavPanel', 'Sound', 'StatusBar', 'Stereo3D', 'Stereo3DCameraOffset', 'Stereo3DHIT', 'ToolBar', 'Textures', 'Transparency', 'Triad', 'Wireframe', 'NavZones', 'NavMode', 'NavSpeed', 'CaptureFileFormat', 'CaptureFileName', 'Record2DCompressMethod', 'Record2DCompressQuality', 'Record2D', 'Record2DFileName', 'Record2DFPS'; [5.0000000000000000e+00   9.2000000000000000e+01   5.7600000000000000e+02   3.5000000000000000e+02], 'CubeSat Orbit Animation', 'NorthPole', 'on', [0.0000000000000000e+00   0.0000000000000000e+00  -1.0000000000000000e+00], [0.0000000000000000e+00   0.0000000000000000e+00   0.0000000000000000e+00], [0.0000000000000000e+00   1.0000000000000000e+00   0.0000000000000000e+00], [1.0000000000000000e+00], 'on', 'on', 'on', 'halfbar', 'on', 'on', 'off', [1.0000000149011612e-01], [0.0000000000000000e+00], 'on', 'on', 'on', 'none', 'off', 'off', 'examine', 'normal', 'tif', '%f_anim_%n.tif', 'auto', [7.5000000000000000e+01], 'off', '%f_anim_%n.avi', 'auto'}"
  m to VRML : Gain  Gain=1e-6
  wires:
  Bus Element In2/1 -> Quaternion to VRML/1(q), Quaternion Inverse/1, Quaternion Inverse1/1
  Constant3/1 -> Radar on/off/1(NavMode)
  Bus Element In3/1 -> Sat Position to VRML/1(x), Sum/1
  Quaternion Inverse/1 -> Quaternion Rotation/1
  Sum/1 -> Antenna Position to VRML/1(x)
  Quaternion Rotation/1 -> Sum/2
  Quaternion Rotation2/1 -> Sun Position to VRML/1(x), Quaternion between r_a and r_b/2
  Quaternion Rotation1/1 -> Quaternion Rotation2/2
  Quaternion Inverse1/1 -> Quaternion Rotation2/1
  Sun Position to VRML/1(xVRML) -> KeepSunInView/1
  Quaternion between r_a and r_b/1 -> Quaternion to VRML1/1(q)
  Constant5/1 -> Quaternion between r_a and r_b/1
  m to VRML/1 -> VR Sink/6
  Antenna Position to VRML/1(xVRML) -> Rate Transition5/1
  Compute Earth Rotation Rate/1(VRMLRot) -> Rate Transition7/1
  Sat Position to VRML/1(xVRML) -> Rate Transition3/1
  Radar on/off/1(Radar) -> VR Sink/8
  Quaternion to VRML1/1(axis_angle) -> Rate Transition2/1
  KeepSunInView/1 -> Compute Umbra Translation/1(I), Rate Transition1/1
  Compute Umbra Translation/1(O) -> Rate Transition4/1
  Satellite Model Scaling/1(Out1) -> VR Sink/3, Compute Antenna Properties/1(SatScale)
  Compute Antenna Properties/1(AntennaScale) -> m to VRML/1
  Compute Antenna Properties/2(AntennaTrans) -> Quaternion Rotation/2
  Bus Element In4/1 -> Quaternion Rotation1/1
  Bus Element In/1 -> Quaternion Rotation1/2
  Rate Transition4/1 -> VR Sink/11
  Rate Transition1/1 -> VR Sink/9
  Rate Transition2/1 -> VR Sink/10
  Bus Element In1/1 -> Compute Earth Rotation Rate/1(EarthRot)
  Rate Transition7/1 -> VR Sink/1
  Rate Transition3/1 -> VR Sink/4
  Rate Transition5/1 -> VR Sink/7
  Quaternion to VRML/1(axis_angle) -> Rate Transition6/1
  Rate Transition6/1 -> VR Sink/5, VR Sink/2

== system asbCubeSat/External Forces and Torques/Perturbations Due to Atmospheric Drag/NRLMSISE-00 Atmosphere Model ==
  "lat, lon, alt" : Inport
  year : Inport  Port=2
  doy : Inport  Port=3
  second : Inport  Port=4
  NRLMSISE-00 Atmosphere Model : aerolibatmos2/NRLMSISE-00 Atmosphere Model  units=Metric (MKS)  lst_input=off  flux_ap_input=off  flags_input=Internal  flags=ones(1,23)  oxygen_in=on  action=Warning
      settings: SourceProductBaseCode=AE
  Subsystem : Subsystem
  Terminator3 : Terminator
  Total mass density : Outport
  wires:
  doy/1 -> NRLMSISE-00 Atmosphere Model/3
  NRLMSISE-00 Atmosphere Model/1 -> Terminator3/1
  year/1 -> NRLMSISE-00 Atmosphere Model/2
  Subsystem/1(Total mass density) -> Total mass density/1
  second/1 -> NRLMSISE-00 Atmosphere Model/4
  NRLMSISE-00 Atmosphere Model/2 -> Subsystem/1(In1)
  "lat, lon, alt"/1 -> NRLMSISE-00 Atmosphere Model/1

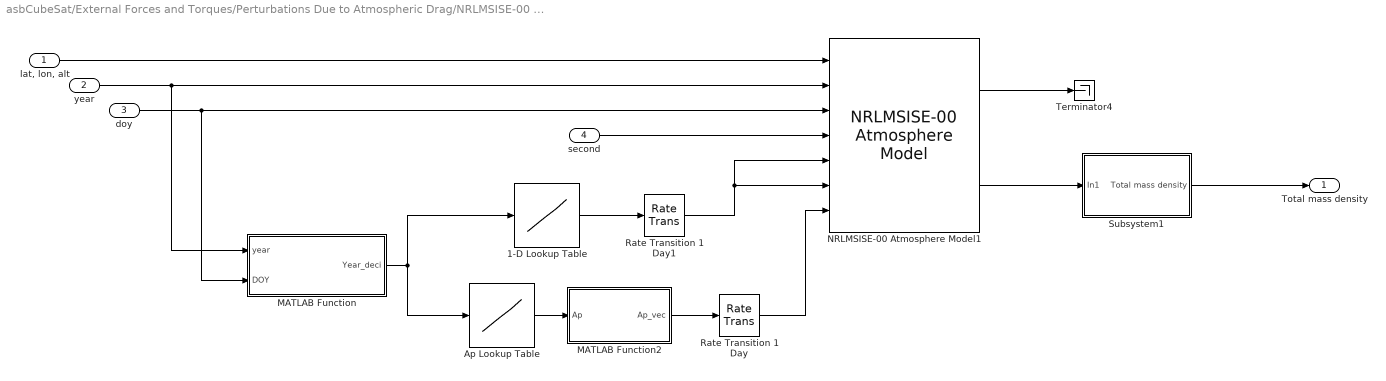
== system asbCubeSat/External Forces and Torques/Perturbations Due to Atmospheric Drag/NRLMSISE-00 Atmosphere Model Solar ==
  "lat, lon, alt" : Inport
  year : Inport  Port=2
  doy : Inport  Port=3
  second : Inport  Port=4
  1-D Lookup Table : Lookup_n-D  NumberOfTableDimensions=1  BreakpointsForDimension1=Solar_Activity(:,1)  Table=Solar_Activity(:,2)  InternalRulePriority=Speed  RndMeth=Simplest  InputSameDT=on
  Ap Lookup Table : Lookup_n-D  NumberOfTableDimensions=1  BreakpointsForDimension1=Solar_Activity(:,1)  Table=Solar_Activity(:,3)  InternalRulePriority=Speed  RndMeth=Simplest  InputSameDT=on
  MATLAB Function : MATLAB Function  TreatAsAtomicUnit=on
  MATLAB Function2 : MATLAB Function  TreatAsAtomicUnit=on
  NRLMSISE-00 Atmosphere Model1 : aerolibatmos2/NRLMSISE-00 Atmosphere Model  units=Metric (MKS)  lst_input=off  flux_ap_input=on  flags_input=Internal  flags=ones(1,23)  oxygen_in=off  action=Warning
      settings: SourceProductBaseCode=AE
  Rate Transition 1 Day : RateTransition  OutPortSampleTime=86400*1
  Rate Transition 1 Day1 : RateTransition  OutPortSampleTime=86400*1
  Subsystem1 : Subsystem
  Terminator4 : Terminator
  Total mass density : Outport
  wires:
  MATLAB Function/1(Year_deci) -> Ap Lookup Table/1, 1-D Lookup Table/1
  second/1 -> NRLMSISE-00 Atmosphere Model1/4
  doy/1 -> MATLAB Function/2(DOY), NRLMSISE-00 Atmosphere Model1/3
  Ap Lookup Table/1 -> MATLAB Function2/1(Ap)
  1-D Lookup Table/1 -> Rate Transition 1 Day1/1
  "lat, lon, alt"/1 -> NRLMSISE-00 Atmosphere Model1/1
  NRLMSISE-00 Atmosphere Model1/2 -> Subsystem1/1(In1)
  MATLAB Function2/1(Ap_vec) -> Rate Transition 1 Day/1
  NRLMSISE-00 Atmosphere Model1/1 -> Terminator4/1
  year/1 -> MATLAB Function/1(year), NRLMSISE-00 Atmosphere Model1/2
  Subsystem1/1(Total mass density) -> Total mass density/1
  Rate Transition 1 Day/1 -> NRLMSISE-00 Atmosphere Model1/7
  Rate Transition 1 Day1/1 -> NRLMSISE-00 Atmosphere Model1/5, NRLMSISE-00 Atmosphere Model1/6

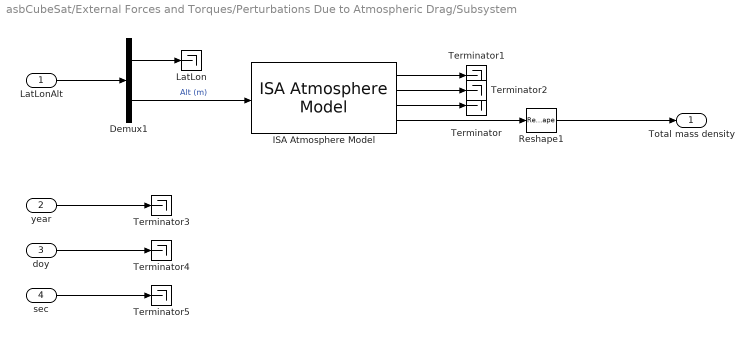
== system asbCubeSat/External Forces and Torques/Perturbations Due to Atmospheric Drag/Subsystem ==
  LatLonAlt : Inport
  year : Inport  Port=2
  doy : Inport  Port=3
  sec : Inport  Port=4
  Demux1 : Demux  Outputs=[2 1]
  ISA Atmosphere Model : aerolibatmos2/ISA Atmosphere Model  custom=off  g=9.80665  gamma=1.4  R=287.0531  L=0.0065  h_trop=11000  h_strat=20000  rho0=1.225  P0=101325  T0=288.15  h0=0
  LatLon : Terminator
  Reshape1 : Reshape
  Terminator{,1..5} (6 alike) : Terminator
  Total mass density : Outport
  wires:
  Demux1/1 -> LatLon/1
  ISA Atmosphere Model/1 -> Terminator1/1
  ISA Atmosphere Model/2 -> Terminator2/1
  ISA Atmosphere Model/3 -> Terminator/1
  Reshape1/1 -> Total mass density/1
  ISA Atmosphere Model/4 -> Reshape1/1
  Demux1/2 -> ISA Atmosphere Model/1  "Alt (m)"
  LatLonAlt/1 -> Demux1/1
  year/1 -> Terminator3/1
  doy/1 -> Terminator4/1
  sec/1 -> Terminator5/1

== system asbCubeSat/External Forces and Torques/Perturbations Due to Atmospheric Drag/Subsystem3 ==
  LatLonAlt : Inport
  year : Inport  Port=2
  doy : Inport  Port=3
  second : Inport  Port=4
  ISA : Subsystem  VariantControl=1
  NRLMSISE-00 Atmosphere Model : Subsystem  VariantControl=2
  NRLMSISE-00 Atmosphere Model Solar : Subsystem  VariantControl=3
  No Drag : Subsystem  VariantControl=0
  Total mass density : Outport

== system asbCubeSat/Visualization/Virtual Reality World/Antenna Position to VRML ==
  x : Inport
  ECEF to VRML : Subsystem
  Length Conversion : aerolibconvert2/Length Conversion  IU=m  OU=km
  km to VRML units : Gain  Gain=1/1000
  xVRML : Outport  VectorParamsAs1DForOutWhenUnconnected=off
  wires:
  Length Conversion/1 -> km to VRML units/1
  km to VRML units/1 -> ECEF to VRML/1(M)
  x/1 -> Length Conversion/1
  ECEF to VRML/1(VR) -> xVRML/1

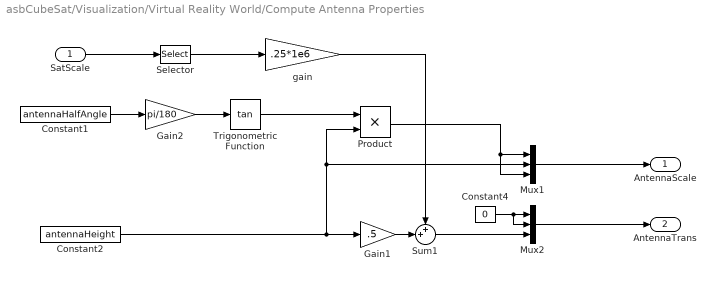
== system asbCubeSat/Visualization/Virtual Reality World/Compute Antenna Properties ==
  SatScale : Inport
  Constant1 : Constant  Value=antennaHalfAngle
  Constant2 : Constant  Value=antennaHeight
  Constant4 : Constant  Value=0
  Gain1 : Gain  Gain=.5
  Gain2 : Gain  Gain=pi/180
  Mux1 : Mux  Inputs=3
  Mux2 : Mux  Inputs=3
  Product : Product
  Selector : Selector  InputPortWidth=3  IndexOptions=Index vector (dialog)  Indices=1  OutputSizes=1
  Sum1 : Sum  Inputs=++|
  Trigonometric Function : Trigonometry  Operator=tan
  gain : Gain  Gain=.25*1e6
  AntennaScale : Outport  VectorParamsAs1DForOutWhenUnconnected=off
  AntennaTrans : Outport  Port=2  VectorParamsAs1DForOutWhenUnconnected=off
  wires:
  Gain2/1 -> Trigonometric Function/1
  Constant4/1 -> Mux2/1, Mux2/2
  Sum1/1 -> Mux2/3
  Constant2/1 -> Gain1/1, Mux1/2, Product/2
  gain/1 -> Sum1/1
  Constant1/1 -> Gain2/1
  Product/1 -> Mux1/3, Mux1/1
  Gain1/1 -> Sum1/2
  Trigonometric Function/1 -> Product/1
  Mux2/1 -> AntennaTrans/1
  Mux1/1 -> AntennaScale/1
  SatScale/1 -> Selector/1
  Selector/1 -> gain/1

== system asbCubeSat/Visualization/Virtual Reality World/Compute Earth Rotation Rate ==
  EarthRot : Inport
  Constant : Constant  Value=0
  Constant1 : Constant  Value=0
  Euler Angles to Quaternions : aerolibobsolete/Euler Angles to Quaternions
      settings: SourceProductBaseCode=AE
  Quaternion to VRML : Subsystem
  Sum : Sum  Inputs=|++
  Unit Delay : UnitDelay  SampleTime=-1  HasFrameUpgradeWarning=on
  Vector Concatenate : Concatenate  NumInputs=3
  VRMLRot : Outport  VectorParamsAs1DForOutWhenUnconnected=off
  wires:
  EarthRot/1 -> Sum/1
  Unit Delay/1 -> Sum/2
  Sum/1 -> Vector Concatenate/3, Unit Delay/1
  Constant/1 -> Vector Concatenate/1
  Constant1/1 -> Vector Concatenate/2
  Vector Concatenate/1 -> Euler Angles to Quaternions/1
  Euler Angles to Quaternions/1 -> Quaternion to VRML/1(q)
  Quaternion to VRML/1(AxisAngle) -> VRMLRot/1

== system asbCubeSat/Visualization/Virtual Reality World/Compute Umbra Translation ==
  I : Inport
  Add : Sum
  ConeHalfLength : Gain  Gain=692
  InvertSunPosECEF : Gain  Gain=-1
  unitVec : Subsystem
  O : Outport  VectorParamsAs1DForOutWhenUnconnected=off
  wires:
  ConeHalfLength/1 -> Add/2
  I/1 -> InvertSunPosECEF/1
  Add/1 -> O/1
  InvertSunPosECEF/1 -> unitVec/1(I), Add/1
  unitVec/1(O) -> ConeHalfLength/1

== system asbCubeSat/Visualization/Virtual Reality World/Quaternion to VRML ==
  q : Inport
  Demux : Demux
  Flip 180 deg : Constant  Value=[0 0 1 0]
  Gain : Gain  Gain=2
  Mux : Mux
  Quaternion Multiplication : aerolibutil/Quaternion Multiplication
  Selector : Selector  InputPortWidth=4  IndexOptions=Index vector (dialog)  Indices=[3 4 2 1]  OutputSizes=1
  Trigonometric Function : Trigonometry  Operator=acos
  axis_angle : Outport  VectorParamsAs1DForOutWhenUnconnected=off
  wires:
  Demux/4 -> Mux/4
  Demux/3 -> Mux/3
  Demux/2 -> Mux/2
  Gain/1 -> Mux/1
  Selector/1 -> axis_angle/1
  q/1 -> Quaternion Multiplication/1
  Mux/1 -> Selector/1
  Trigonometric Function/1 -> Gain/1
  Demux/1 -> Trigonometric Function/1
  Flip 180 deg/1 -> Quaternion Multiplication/2
  Quaternion Multiplication/1 -> Demux/1

== system asbCubeSat/Visualization/Virtual Reality World/Quaternion to VRML1 ==
  q : Inport
  Demux : Demux
  Flip 180 deg : Constant  Value=[0 0 1 0]
  Gain : Gain  Gain=2
  Mux : Mux
  Quaternion Multiplication : aerolibutil/Quaternion Multiplication
  Selector : Selector  InputPortWidth=4  IndexOptions=Index vector (dialog)  Indices=[3 4 2 1]  OutputSizes=1
  Trigonometric Function : Trigonometry  Operator=acos
  axis_angle : Outport  VectorParamsAs1DForOutWhenUnconnected=off
  wires:
  Demux/4 -> Mux/4
  Demux/3 -> Mux/3
  Demux/2 -> Mux/2
  Gain/1 -> Mux/1
  Selector/1 -> axis_angle/1
  Mux/1 -> Selector/1
  Trigonometric Function/1 -> Gain/1
  Demux/1 -> Trigonometric Function/1
  Flip 180 deg/1 -> Quaternion Multiplication/2
  q/1 -> Quaternion Multiplication/1
  Quaternion Multiplication/1 -> Demux/1

== system asbCubeSat/Visualization/Virtual Reality World/Radar on//off ==
  NavMode : Inport
  Add : Sum  Inputs=-+
  Compare To Constant : simulink/Logic and Bit Operations/Compare To Constant  relop===  const=1  OutDataTypeStr=boolean  ZeroCross=off
  Constant : Constant
  Data Type Conversion : DataTypeConversion  OutDataTypeStr=double
  Gain : Gain  Gain=0.6
  Radar : Outport  VectorParamsAs1DForOutWhenUnconnected=off
  wires:
  NavMode/1 -> Compare To Constant/1
  Compare To Constant/1 -> Data Type Conversion/1
  Data Type Conversion/1 -> Gain/1
  Gain/1 -> Add/1
  Constant/1 -> Add/2
  Add/1 -> Radar/1

== system asbCubeSat/Visualization/Virtual Reality World/Sat Position to VRML ==
  x : Inport
  ECEF to VRML : Subsystem
  Length Conversion : aerolibconvert2/Length Conversion  IU=m  OU=km
  km to VRML units : Gain  Gain=1/1000
  xVRML : Outport  VectorParamsAs1DForOutWhenUnconnected=off
  wires:
  ECEF to VRML/1(VR) -> xVRML/1
  x/1 -> Length Conversion/1
  km to VRML units/1 -> ECEF to VRML/1(M)
  Length Conversion/1 -> km to VRML units/1

== system asbCubeSat/Visualization/Virtual Reality World/Satellite Model Scaling ==
  Constant : Constant  Value=cubesatSize
  Mux : Mux  Inputs=3
  ScaleModelToVRML : Gain  Gain=1/.3e6
  Out1 : Outport  VectorParamsAs1DForOutWhenUnconnected=off
  wires:
  ScaleModelToVRML/1 -> Mux/3, Mux/1, Mux/2
  Constant/1 -> ScaleModelToVRML/1
  Mux/1 -> Out1/1

== system asbCubeSat/Visualization/Virtual Reality World/Sun Position to VRML ==
  x : Inport
  ECEF to VRML : Subsystem
  Length Conversion : aerolibconvert2/Length Conversion  IU=m  OU=km
  km to VRML units : Gain  Gain=1/1000
  xVRML : Outport  VectorParamsAs1DForOutWhenUnconnected=off
  wires:
  ECEF to VRML/1(VR) -> xVRML/1
  x/1 -> Length Conversion/1
  km to VRML units/1 -> ECEF to VRML/1(M)
  Length Conversion/1 -> km to VRML units/1

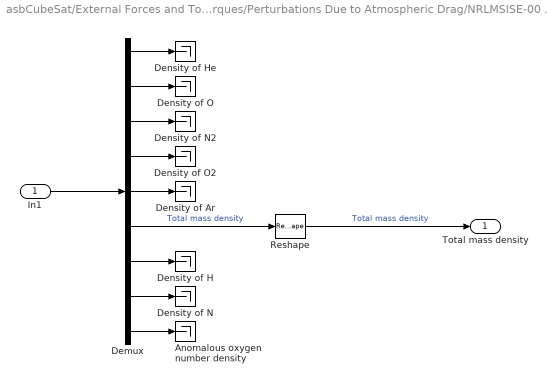
== system asbCubeSat/External Forces and Torques/Perturbations Due to Atmospheric Drag/NRLMSISE-00 Atmosphere Model/Subsystem ==
  In1 : Inport
  Anomalous oxygen number density : Terminator
  Demux : Demux  Outputs=9
  Density of Ar : Terminator
  Density of H : Terminator
  Density of He : Terminator
  Density of N : Terminator
  Density of N2 : Terminator
  Density of O : Terminator
  Density of O2 : Terminator
  Reshape : Reshape
  Total mass density : Outport
  wires:
  Demux/5 -> Density of Ar/1
  Demux/2 -> Density of O/1
  Demux/1 -> Density of He/1
  Demux/7 -> Density of H/1
  Demux/8 -> Density of N/1
  Demux/3 -> Density of N2/1
  Demux/9 -> Anomalous oxygen number density/1
  Demux/4 -> Density of O2/1
  In1/1 -> Demux/1
  Demux/6 -> Reshape/1  "Total mass density"
  Reshape/1 -> Total mass density/1  "Total mass density"

== system asbCubeSat/External Forces and Torques/Perturbations Due to Atmospheric Drag/NRLMSISE-00 Atmosphere Model Solar/Subsystem1 ==
  In1 : Inport
  Anomalous oxygen number density : Terminator
  Demux : Demux  Outputs=9
  Density of Ar : Terminator
  Density of H : Terminator
  Density of He : Terminator
  Density of N : Terminator
  Density of N2 : Terminator
  Density of O : Terminator
  Density of O2 : Terminator
  Reshape3 : Reshape
  Total mass density : Outport
  wires:
  Demux/5 -> Density of Ar/1
  Demux/2 -> Density of O/1
  Demux/1 -> Density of He/1
  Demux/7 -> Density of H/1
  Demux/8 -> Density of N/1
  Demux/3 -> Density of N2/1
  Demux/9 -> Anomalous oxygen number density/1
  Demux/4 -> Density of O2/1
  In1/1 -> Demux/1
  Demux/6 -> Reshape3/1  "Total mass density"
  Reshape3/1 -> Total mass density/1  "Total mass density"

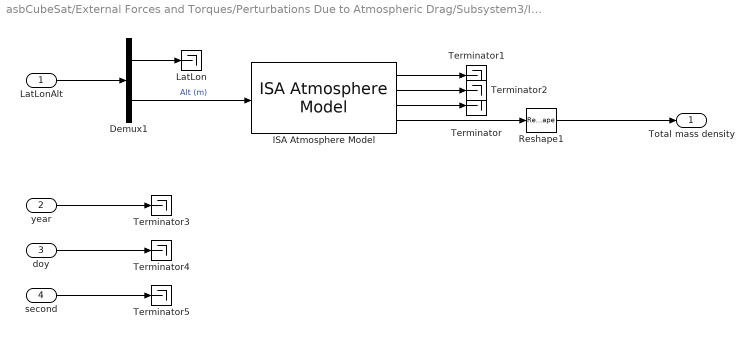
== system asbCubeSat/External Forces and Torques/Perturbations Due to Atmospheric Drag/Subsystem3/ISA ==
  LatLonAlt : Inport
  year : Inport  Port=2
  doy : Inport  Port=3
  second : Inport  Port=4
  Demux1 : Demux  Outputs=[2 1]
  ISA Atmosphere Model : aerolibatmos2/ISA Atmosphere Model  custom=off  g=9.80665  gamma=1.4  R=287.0531  L=0.0065  h_trop=11000  h_strat=20000  rho0=1.225  P0=101325  T0=288.15  h0=0
  LatLon : Terminator
  Reshape1 : Reshape
  Terminator{,1..5} (6 alike) : Terminator
  Total mass density : Outport
  wires:
  Demux1/1 -> LatLon/1
  ISA Atmosphere Model/1 -> Terminator1/1
  ISA Atmosphere Model/2 -> Terminator2/1
  ISA Atmosphere Model/3 -> Terminator/1
  Reshape1/1 -> Total mass density/1
  ISA Atmosphere Model/4 -> Reshape1/1
  Demux1/2 -> ISA Atmosphere Model/1  "Alt (m)"
  LatLonAlt/1 -> Demux1/1
  year/1 -> Terminator3/1
  doy/1 -> Terminator4/1
  second/1 -> Terminator5/1

== system asbCubeSat/External Forces and Torques/Perturbations Due to Atmospheric Drag/Subsystem3/NRLMSISE-00 Atmosphere Model ==
  LatLonAlt : Inport
  year : Inport  Port=2
  doy : Inport  Port=3
  second : Inport  Port=4
  NRLMSISE-00 Atmosphere Model : aerolibatmos2/NRLMSISE-00 Atmosphere Model  units=Metric (MKS)  lst_input=off  flux_ap_input=off  flags_input=Internal  flags=ones(1,23)  oxygen_in=on  action=Warning
      settings: SourceProductBaseCode=AE
  Subsystem : Subsystem
  Terminator3 : Terminator
  Total mass density : Outport
  wires:
  doy/1 -> NRLMSISE-00 Atmosphere Model/3
  NRLMSISE-00 Atmosphere Model/1 -> Terminator3/1
  year/1 -> NRLMSISE-00 Atmosphere Model/2
  Subsystem/1(Total mass density) -> Total mass density/1
  second/1 -> NRLMSISE-00 Atmosphere Model/4
  NRLMSISE-00 Atmosphere Model/2 -> Subsystem/1(In1)
  LatLonAlt/1 -> NRLMSISE-00 Atmosphere Model/1

== system asbCubeSat/External Forces and Torques/Perturbations Due to Atmospheric Drag/Subsystem3/NRLMSISE-00 Atmosphere Model Solar ==
  LatLonAlt : Inport
  year : Inport  Port=2
  doy : Inport  Port=3
  second : Inport  Port=4
  NRLMSISE-00 Atmosphere Model1 : aerolibatmos2/NRLMSISE-00 Atmosphere Model  units=Metric (MKS)  lst_input=off  flux_ap_input=on  flags_input=Internal  flags=ones(1,23)  oxygen_in=off  action=Warning
      settings: SourceProductBaseCode=AE
  Rate Transition 1 Day : RateTransition
  Rate Transition 1 Day1 : RateTransition
  Subsystem : Subsystem  TreatAsAtomicUnit=on  SystemSampleTime=86400*1
  Subsystem1 : Subsystem
  Terminator4 : Terminator
  Total mass density : Outport
  wires:
  second/1 -> NRLMSISE-00 Atmosphere Model1/4
  doy/1 -> Subsystem/2(DOY), NRLMSISE-00 Atmosphere Model1/3
  LatLonAlt/1 -> NRLMSISE-00 Atmosphere Model1/1
  NRLMSISE-00 Atmosphere Model1/2 -> Subsystem1/1(In1)
  NRLMSISE-00 Atmosphere Model1/1 -> Terminator4/1
  year/1 -> Subsystem/1(year), NRLMSISE-00 Atmosphere Model1/2
  Subsystem1/1(Total mass density) -> Total mass density/1
  Rate Transition 1 Day/1 -> NRLMSISE-00 Atmosphere Model1/7
  Subsystem/1(Out1) -> Rate Transition 1 Day1/1
  Subsystem/2(Ap_vec) -> Rate Transition 1 Day/1
  Rate Transition 1 Day1/1 -> NRLMSISE-00 Atmosphere Model1/5, NRLMSISE-00 Atmosphere Model1/6

== system asbCubeSat/External Forces and Torques/Perturbations Due to Atmospheric Drag/Subsystem3/No Drag ==
  LatLonAlt : Inport
  year : Inport  Port=2
  doy : Inport  Port=3
  second : Inport  Port=4
  Case 1: No Drag : Constant  Value=0
  Terminator{,1..3} (4 alike) : Terminator
  Total mass density : Outport
  wires:
  Case 1: No Drag/1 -> Total mass density/1
  doy/1 -> Terminator2/1
  year/1 -> Terminator1/1
  LatLonAlt/1 -> Terminator/1
  second/1 -> Terminator3/1

== system asbCubeSat/Visualization/Virtual Reality World/Antenna Position to VRML/ECEF to VRML ==
  M : Inport  PortDimensions=3
  Selector : Selector  InputPortWidth=3  IndexOptions=Index vector (dialog)  Indices=[2 3 1]  OutputSizes=1
  VR : Outport  PortDimensions=3  VectorParamsAs1DForOutWhenUnconnected=off
  wires:
  M/1 -> Selector/1
  Selector/1 -> VR/1
